simulink model "starshotsim_dev"  (R2023a)
settings: Solver=FixedStepAuto  StartTime=0.0  StopTime=350000  FixedStep=0.01  MaxStep=4.0  MinStep=.001  RelTol=1e-6
values from neighbouring files (symbols this model uses):
  B0 = 3.12e-5    (= 3.12e-05)    [starshot_ACS_setup.m]
  G = 6.67e-11    [starshot_ACS_setup.m]
  M_Earth = 5.972e24    (= 5.972e+24)    [starshot_ACS_setup.m]
  q0 = [qmatlab(2:4),qmatlab(1)]'    [starshot_ACS_setup.m]
  R_Earth = 6.378e6    (= 6378000)    [starshot_ACS_setup.m]
undefined symbols (not defined in the file or in its folder): DiscIntNeverNeededParam, starshot
libraries: simulink x3, dspmathops x3, vrlib x2, sharedtransform x1
(part 1 of 2)
settings Model: SimulationMode=accelerator  Creator=armen  LastModifiedBy=SSDS_1
settings SolverCC: AlgebraicLoopSolver=TrustRegion
settings DataIOCC: ReturnWorkspaceOutputs=off
settings OptimizationCC: DefaultParameterBehavior=Inlined  UseDivisionForNetSlopeComputation=on  UseFloatMulNetSlope=on  InlineInvariantSignals=on  PassReuseOutputArgsAs=Individual arguments  ZeroExternalMemoryAtStartup=off  ZeroInternalMemoryAtStartup=off  NoFixptDivByZeroProtection=on  EfficientFloat2IntCast=on  LifeSpan=1  EfficientTunableParamExpr=on
settings DebuggingCC: ParameterTunabilityLossMsg=error  UnconnectedInputMsg=warning  UnconnectedOutputMsg=warning  UnconnectedLineMsg=warning  ArithmeticOperatorsInVariantConditions=warning
settings HardwareCC: ProdBitPerPointer=32  ProdBitPerSizeT=32  ProdBitPerPtrDiffT=32  ProdLargestAtomicInteger=Long  ProdLargestAtomicFloat=Double  ProdWordSize=32  ProdHWDeviceType=ARM Compatible->ARM Cortex
settings ModelReferenceCC: EnableRefExpFcnMdlSchedulingChecks=on
settings SFSimCC: SimUseLocalCustomCode=off  MATLABDynamicMemAlloc=off  CustomCodeUndefinedFunction=UseInterfaceOnly  SimTargetLang=C++
settings RTWCC: Description=Embedded Coder  SystemTargetFile=ert.tlc  GenCodeOnly=on  TemplateMakefile=ert_default_tmf  GenerateReport=on  RTWUseLocalCustomCode=off  IncludeHyperlinkInReport=on  LaunchReport=on  TargetLang=C++  GenerateTraceInfo=on  GenerateTraceReport=on  GenerateTraceReportSl=on  GenerateTraceReportSf=on  GenerateTraceReportEml=on
settings CodeAppCC: ForceParamTrailComments=on  IgnoreCustomStorageClasses=off  OperatorAnnotations=on  SimulinkDataObjDesc=on  SFDataObjDesc=on  MATLABFcnDesc=on  CustomSymbolStrGlobalVar=rt$N$M  CustomSymbolStrType=$N$M  CustomSymbolStrFcn=$N$M$F  CustomSymbolStrMacro=$N$M  InsertBlockDesc=on  StateflowObjectComments=on  MATLABSourceComments=on
settings ERTTargetCC: TargetLangStandard=C++03 (ISO)  GenerateSampleERTMain=on  IncludeMdlTerminateFcn=off  CombineSignalStateStructs=on  SupportAbsoluteTime=off  CodeInterfacePackaging=C++ class  SupportComplex=off  SupportNonInlinedSFcns=on  InlinedParameterPlacement=NonHierarchical  RootIOFormat=Structure reference  ERTCustomFileTemplate=example_file_process.tlc  ERTFilePackagingFormat=CompactWithDataFile

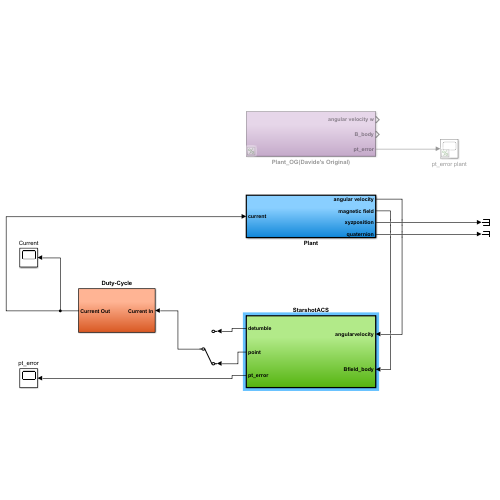
[thumbnail: Simulink's stored preview of the top-level diagram]
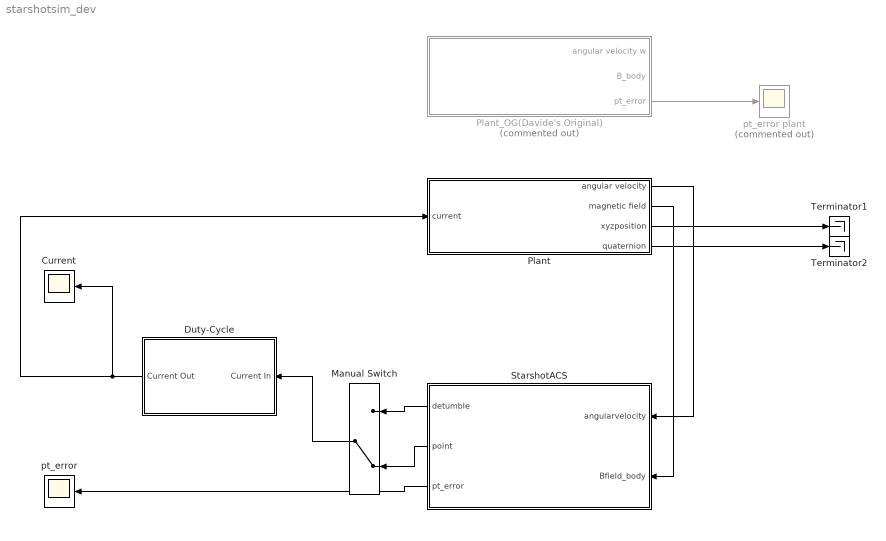
== system starshotsim_dev ==
  Current : Scope
  Duty-Cycle : Subsystem
  Manual Switch : ManualSwitch  CurrentSetting=0
  Plant : Subsystem  TreatAsAtomicUnit=on
  Plant_OG(Davide's Original) : Subsystem  Commented=on
  StarshotACS : Subsystem  TreatAsAtomicUnit=on  SystemSampleTime=0.2
  Terminator1 : Terminator
  Terminator2 : Terminator
  pt_error : Scope
  pt_error plant : Scope  Commented=on
  wires:
  StarshotACS/1(detumble) -> Manual Switch/1
  Plant/4(quaternion) -> Terminator2/1
  Plant/3(xyzposition) -> Terminator1/1
  Plant_OG(Davide's Original)/3(pt_error) -> pt_error plant/1
  StarshotACS/2(point) -> Manual Switch/2
  Plant/1(angular velocity) -> StarshotACS/1(angularvelocity)
  Plant/2(magnetic field) -> StarshotACS/2(Bfield_body)
  Manual Switch/1 -> Duty-Cycle/1(Current In)
  StarshotACS/3(pt_error) -> pt_error/1
  Duty-Cycle/1(Current Out) -> Current/1, Plant/1(current)

== system starshotsim_dev/Duty-Cycle ==
  Current In : Inport
  Demux1 : Demux  Outputs=3
  Duty-cycle input : Constant  Value=starshot.controller.dutyclc
  Mux3 : Mux  Inputs=3
  PWM1 : simulink/Discontinuities/PWM  DisableCoverage=on  Period=starshot.controller.dutyT  InitialDelay=0  DisallowZeroDutyCycle=off  RunAtFixedTimeIntervals=on  SampleTime=0.2
  Product : Product
  Current Out : Outport
  wires:
  Demux1/2 -> Mux3/2
  Demux1/1 -> Mux3/1
  PWM1/1 -> Product/2
  Demux1/3 -> Product/1
  Product/1 -> Mux3/3
  Mux3/1 -> Current Out/1
  Current In/1 -> Demux1/1
  Duty-cycle input/1 -> PWM1/1

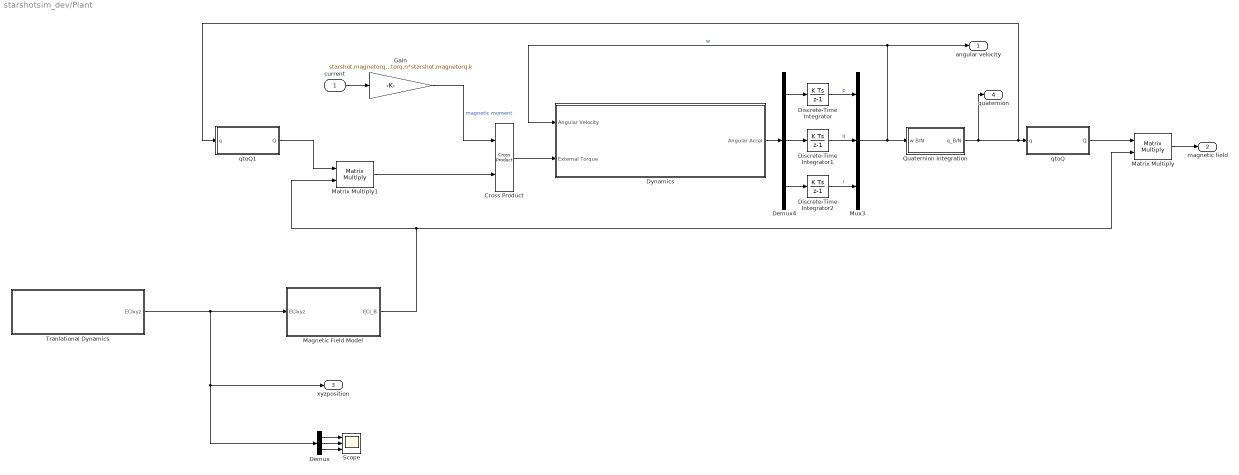
== system starshotsim_dev/Plant ==
  current : Inport
  Cross Product : vrlib/Utilities/Cross Product
  Demux : Demux  Outputs=3
  Demux4 : Demux  Outputs=3
  Discrete-Time Integrator : DiscreteIntegrator  InitialCondition=starshot.IC.w(1)  SampleTime=-1  ICPrevOutput=DiscIntNeverNeededParam  ICPrevScaledInput=DiscIntNeverNeededParam
  Discrete-Time Integrator1 : DiscreteIntegrator  InitialCondition=starshot.IC.w(2)  SampleTime=-1  ICPrevOutput=DiscIntNeverNeededParam  ICPrevScaledInput=DiscIntNeverNeededParam
  Discrete-Time Integrator2 : DiscreteIntegrator  InitialCondition=starshot.IC.w(3)  SampleTime=-1  ICPrevOutput=DiscIntNeverNeededParam  ICPrevScaledInput=DiscIntNeverNeededParam
  Dynamics : Subsystem  TreatAsAtomicUnit=on
  Gain : Gain  Gain=starshot.magnetorq.A*starshot.magnetorq.n*starshot.magnetorq.k
  Magnetic Field Model : Subsystem  TreatAsAtomicUnit=on
  Matrix Multiply : Product  Multiplication=Matrix(*)
  Matrix Multiply1 : Product  Multiplication=Matrix(*)
  Mux3 : Mux  Inputs=3
  Quaternion Integration : Subsystem
  Scope : Scope  NumInputPorts=3
  Tranlational Dynamics : Subsystem  TreatAsAtomicUnit=on
  qtoQ : Subsystem  TreatAsAtomicUnit=on
  qtoQ1 : Subsystem  TreatAsAtomicUnit=on
  angular velocity : Outport
  magnetic field : Outport  Port=2
  xyzposition : Outport  Port=3
  quaternion : Outport  Port=4
  wires:
  Matrix Multiply/1 -> magnetic field/1
  Magnetic Field Model/1(ECI_B) -> Matrix Multiply/2, Matrix Multiply1/2
  Discrete-Time Integrator1/1 -> Mux3/2  "q"
  Discrete-Time Integrator2/1 -> Mux3/3  "r"
  Demux4/3 -> Discrete-Time Integrator2/1
  Demux4/1 -> Discrete-Time Integrator/1
  Tranlational Dynamics/1(ECIxyz) -> Demux/1, xyzposition/1, Magnetic Field Model/1(ECIxyz)
  Quaternion Integration/1(q_B/N) -> qtoQ1/1(q), qtoQ/1(q), quaternion/1
  Dynamics/1(Angular Accel) -> Demux4/1
  Mux3/1 -> Quaternion Integration/1(w B/N), Dynamics/1(Angular Velocity), angular velocity/1  "w"
  current/1 -> Gain/1
  Gain/1 -> Cross Product/1  "magnetic moment"
  Cross Product/1 -> Dynamics/2(External Torque)
  Discrete-Time Integrator/1 -> Mux3/1  "p"
  Demux4/2 -> Discrete-Time Integrator1/1
  Demux/2 -> Scope/2
  Demux/1 -> Scope/1
  Demux/3 -> Scope/3
  qtoQ/1(Q) -> Matrix Multiply/1
  Matrix Multiply1/1 -> Cross Product/2
  qtoQ1/1(Q) -> Matrix Multiply1/1

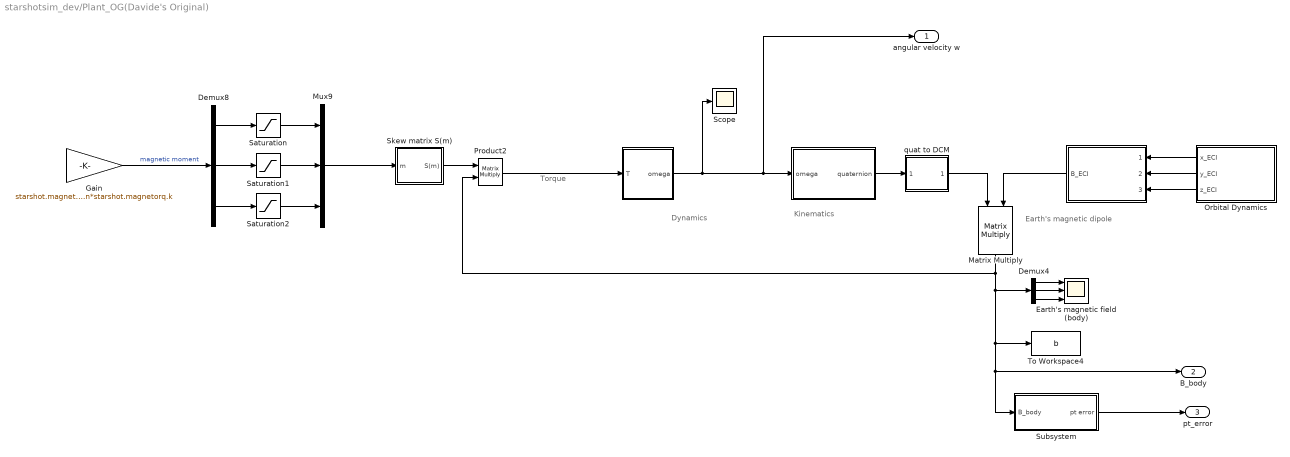
== system starshotsim_dev/Plant_OG(Davide's Original) ==
  note: Torque
  note: Dynamics
  note: Kinematics
  note: Earth's magnetic dipole
  " " : Subsystem
  "   " : Subsystem
  "     " : Subsystem
  Demux4 : Demux  Outputs=3
  Demux8 : Demux  Outputs=3
  Earth's magnetic field (body) : Scope  NumInputPorts=3
  Gain : Gain  Gain=starshot.magnetorq.A*starshot.magnetorq.n*starshot.magnetorq.k
  Matrix Multiply : Product  Multiplication=Matrix(*)
  Mux9 : Mux  Inputs=3
  Orbital Dynamics : Subsystem
  Product2 : Product  Multiplication=Matrix(*)
  Saturation : Saturate  UpperLimit=starshot.magnetorq.m_max_x  LowerLimit=-starshot.magnetorq.m_max_x
  Saturation1 : Saturate  UpperLimit=starshot.magnetorq.m_max_y  LowerLimit=-starshot.magnetorq.m_max_y
  Saturation2 : Saturate  UpperLimit=starshot.magnetorq.m_max_z  LowerLimit=-starshot.magnetorq.m_max_z
  Scope : Scope
  Skew matrix S(m) : Subsystem
  Subsystem : Subsystem
  To Workspace4 : ToWorkspace  VariableName=b  SaveFormat=Timeseries  SampleTime=-1
  quat to DCM : Subsystem  mask(Direction Cosine Matrix){}
      mask help: Determines the 3x3 Direction Cosine Matrix (DCM) from a 4x1 quaternion orientation vector. The outputted DCM transforms vectors from inertial axes to body axes. This version corrects the fucked-up MATLAB one.
      mask Help:
      | <p>This block determines the 3x3 Direction Cosine Matrix (DCM) from a 4x1 quaternion orientation vector. The outputted DCM transforms vectors from inertial axes to body axes.  This version corrects the fucked-up MATLAB one</p>
      | 
      | <p>The block input and output contain more than one signal as described below.</p>
      | 
      | <p><H4>Block Vector Input - Quaternion</H4>
      | <ul>
      | <li>q0</li>
      | <li>q1</li>
      | <li>q2</li>
      | <li>q3</li>
      | </ul>
      | </p>
      | 
      | <p><H4>Block Matrix Output - Direction Cosine Matrix  </H4>
      |     <ul>
      |    </ul>
      |    </p>
      mask Display: disp('q to Q')
  angular velocity w : Outport
  B_body : Outport  Port=2
  pt_error : Outport  Port=3
  wires:
  ? -> Gain/1
  Demux8/2 -> Saturation1/1
  Demux8/1 -> Saturation/1
  Demux8/3 -> Saturation2/1
  Saturation/1 -> Mux9/1
  Saturation1/1 -> Mux9/2
  Saturation2/1 -> Mux9/3
  Mux9/1 -> Skew matrix S(m)/1(m)
  Skew matrix S(m)/1(S(m)) -> Product2/1
  Product2/1 -> "     "/1(T)
  Orbital Dynamics/3(z_ECI) -> " "/3(" ")
  Demux4/3 -> Earth's magnetic field (body)/3
  "   "/1(quaternion) -> quat to DCM/1(e0 e1 e2 e3)
  quat to DCM/1(DCM) -> Matrix Multiply/1
  " "/1(B_ECI) -> Matrix Multiply/2
  Orbital Dynamics/1(x_ECI) -> " "/1(" ")
  Matrix Multiply/1 -> Product2/2, B_body/1, Subsystem/1(B_body), To Workspace4/1, Demux4/1
  Orbital Dynamics/2(y_ECI) -> " "/2(" ")
  Demux4/2 -> Earth's magnetic field (body)/2
  Demux4/1 -> Earth's magnetic field (body)/1
  "     "/1(omega) -> Scope/1, angular velocity w/1, "   "/1(omega)
  Subsystem/1(pt error) -> pt_error/1
  Gain/1 -> Demux8/1  "magnetic moment"

== system starshotsim_dev/StarshotACS ==
  angularvelocity : Inport
  Bfield_body : Inport  Port=2
  KD_controller : Subsystem
  Orientation controller : Subsystem
  Point Error : Subsystem
  detumble : Outport
  point : Outport  Port=2
  pt_error : Outport  Port=3
  wires:
  Bfield_body/1 -> KD_controller/2(B(body)), Point Error/1(B_body), Orientation controller/2(B(body))  "Bfield_body"
  angularvelocity/1 -> Orientation controller/1(Omega), KD_controller/1(Omega)  "angularvelocity"
  Point Error/1(pt error) -> pt_error/1
  KD_controller/1(Current) -> detumble/1
  Orientation controller/1(Current) -> point/1

== system starshotsim_dev/Plant/Dynamics ==
  Angular Velocity : Inport
  External Torque : Inport  Port=2
  Constant : Constant  Value=starshot.IC.massproperties.I
  Constant1 : Constant  Value=starshot.IC.massproperties.Iinv
  Cross Product : vrlib/Utilities/Cross Product
  Product : Product  Multiplication=Matrix(*)
  Product1 : Product  Multiplication=Matrix(*)
  Sum : Sum  Inputs=+-
  Angular Accel : Outport
  wires:
  Angular Velocity/1 -> Cross Product/1, Product/2
  Constant/1 -> Product/1
  Cross Product/1 -> Sum/2
  Product/1 -> Cross Product/2
  External Torque/1 -> Sum/1
  Constant1/1 -> Product1/1
  Product1/1 -> Angular Accel/1
  Sum/1 -> Product1/2

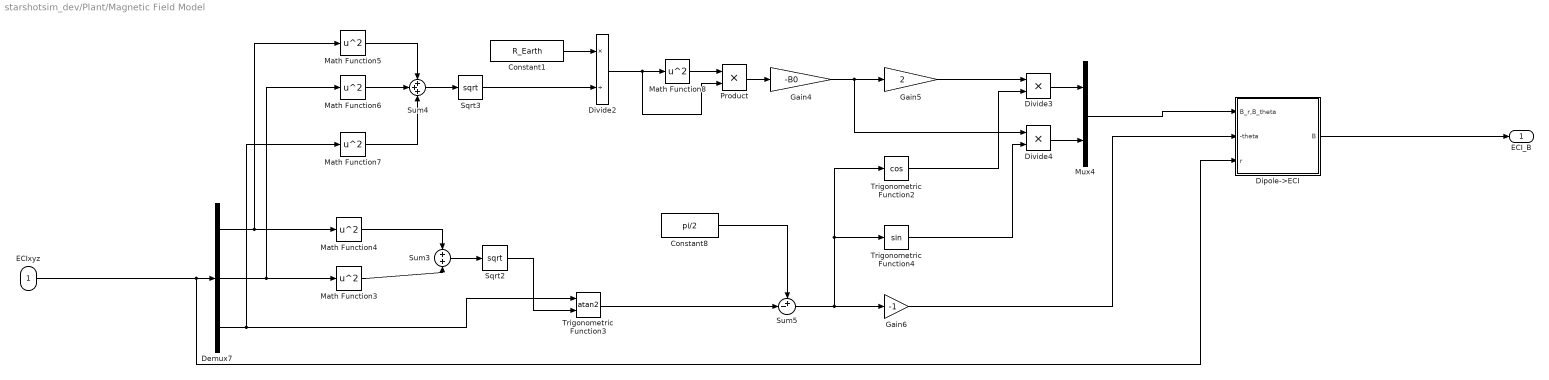
== system starshotsim_dev/Plant/Magnetic Field Model ==
  ECIxyz : Inport
  Constant1 : Constant  Value=R_Earth
  Constant8 : Constant  Value=pi/2
  Demux7 : Demux  Outputs=3
  Dipole->ECI : Subsystem  TreatAsAtomicUnit=on
  Divide2 : Product  Inputs=*/
  Divide3 : Product  Inputs=**
  Divide4 : Product  Inputs=**
  Gain4 : Gain  Gain=-B0
  Gain5 : Gain  Gain=2
  Gain6 : Gain  Gain=-1
  Math Function{3..8} (6 alike) : Math  Operator=square  SignedPower=on
  Mux4 : Mux  Inputs=2
  Product : Product
  Sqrt2 : Sqrt
  Sqrt3 : Sqrt
  Sum3 : Sum
  Sum4 : Sum  Inputs=+++
  Sum5 : Sum  Inputs=+-|
  Trigonometric Function2 : Trigonometry  Operator=cos
  Trigonometric Function3 : Trigonometry  Operator=atan2
  Trigonometric Function4 : Trigonometry
  ECI_B : Outport
  wires:
  Math Function7/1 -> Sum4/3
  Constant1/1 -> Divide2/1
  Math Function5/1 -> Sum4/1
  Math Function4/1 -> Sum3/1
  Demux7/3 -> Math Function7/1, Trigonometric Function3/1
  Sqrt2/1 -> Trigonometric Function3/2
  Product/1 -> Gain4/1
  Math Function8/1 -> Product/1
  Gain5/1 -> Divide3/1
  Sqrt3/1 -> Divide2/2
  Sum4/1 -> Sqrt3/1
  Divide2/1 -> Product/2, Math Function8/1
  Sum3/1 -> Sqrt2/1
  Math Function3/1 -> Sum3/2
  Demux7/1 -> Math Function5/1, Math Function4/1
  Gain4/1 -> Gain5/1, Divide4/1
  Trigonometric Function2/1 -> Divide3/2
  Math Function6/1 -> Sum4/2
  Demux7/2 -> Math Function6/1, Math Function3/1
  Sum5/1 -> Trigonometric Function2/1, Trigonometric Function4/1, Gain6/1
  Trigonometric Function4/1 -> Divide4/2
  Gain6/1 -> Dipole->ECI/2(-theta)
  Divide4/1 -> Mux4/2
  Trigonometric Function3/1 -> Sum5/2
  Constant8/1 -> Sum5/1
  Mux4/1 -> Dipole->ECI/1(B_r,B_theta)
  Dipole->ECI/1(B) -> ECI_B/1
  Divide3/1 -> Mux4/1
  ECIxyz/1 -> Dipole->ECI/3(r), Demux7/1

== system starshotsim_dev/Plant/Quaternion Integration ==
  w B/N : Inport
  Discrete-Time Integrator1 : DiscreteIntegrator  InitialCondition=q0  SampleTime=-1  ICPrevOutput=DiscIntNeverNeededParam  ICPrevScaledInput=DiscIntNeverNeededParam
  q_normalize : Subsystem
  qderiv : Subsystem
  q_B/N : Outport
  wires:
  w B/N/1 -> qderiv/1(w)
  q_normalize/1(q_out) -> qderiv/2(q), q_B/N/1
  Discrete-Time Integrator1/1 -> q_normalize/1(q_in)
  qderiv/1(qd) -> Discrete-Time Integrator1/1

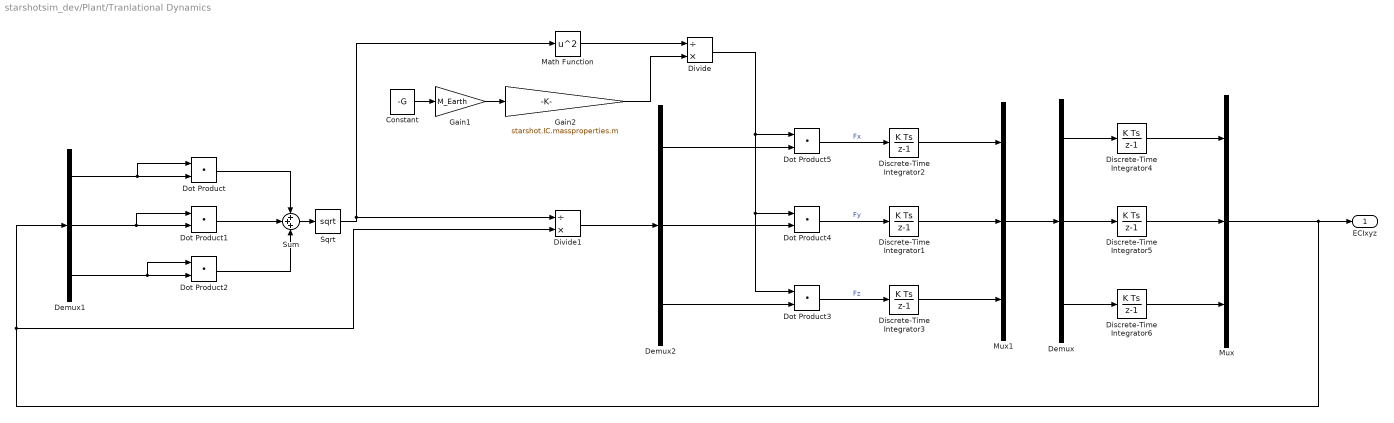
== system starshotsim_dev/Plant/Tranlational Dynamics ==
  Constant : Constant  Value=-G
  Demux : Demux  Outputs=3
  Demux1 : Demux  Outputs=3
  Demux2 : Demux  Outputs=3
  Discrete-Time Integrator1 : DiscreteIntegrator  InitialCondition=starshot.IC.ydot  SampleTime=-1  ICPrevOutput=DiscIntNeverNeededParam  ICPrevScaledInput=DiscIntNeverNeededParam
  Discrete-Time Integrator2 : DiscreteIntegrator  InitialCondition=starshot.IC.xdot  SampleTime=-1  ICPrevOutput=DiscIntNeverNeededParam  ICPrevScaledInput=DiscIntNeverNeededParam
  Discrete-Time Integrator3 : DiscreteIntegrator  InitialCondition=starshot.IC.zdot  SampleTime=-1  ICPrevOutput=DiscIntNeverNeededParam  ICPrevScaledInput=DiscIntNeverNeededParam
  Discrete-Time Integrator4 : DiscreteIntegrator  InitialCondition=starshot.IC.x  SampleTime=-1  ICPrevOutput=DiscIntNeverNeededParam  ICPrevScaledInput=DiscIntNeverNeededParam
  Discrete-Time Integrator5 : DiscreteIntegrator  InitialCondition=starshot.IC.y  SampleTime=-1  ICPrevOutput=DiscIntNeverNeededParam  ICPrevScaledInput=DiscIntNeverNeededParam
  Discrete-Time Integrator6 : DiscreteIntegrator  InitialCondition=starshot.IC.z  SampleTime=-1  ICPrevOutput=DiscIntNeverNeededParam  ICPrevScaledInput=DiscIntNeverNeededParam
  Divide : Product  Inputs=/*
  Divide1 : Product  Inputs=/*
  Dot Product{,1..5} (6 alike) : DotProduct  OutDataTypeStr=Inherit: Inherit via internal rule
  Gain1 : Gain  Gain=M_Earth
  Gain2 : Gain  Gain=starshot.IC.massproperties.m
  Math Function : Math  Operator=square  SignedPower=on
  Mux : Mux  Inputs=3
  Mux1 : Mux  Inputs=3
  Sqrt : Sqrt
  Sum : Sum  Inputs=+++
  ECIxyz : Outport
  wires:
  Discrete-Time Integrator6/1 -> Mux/3
  Discrete-Time Integrator5/1 -> Mux/2
  Discrete-Time Integrator4/1 -> Mux/1
  Demux/3 -> Discrete-Time Integrator6/1
  Demux/1 -> Discrete-Time Integrator4/1
  Mux1/1 -> Demux/1
  Discrete-Time Integrator3/1 -> Mux1/3
  Demux/2 -> Discrete-Time Integrator5/1
  Demux1/2 -> Dot Product1/1, Dot Product1/2
  Sum/1 -> Sqrt/1
  Dot Product4/1 -> Discrete-Time Integrator1/1  "Fy"
  Demux1/1 -> Dot Product/1, Dot Product/2
  Dot Product3/1 -> Discrete-Time Integrator3/1  "Fz"
  Divide/1 -> Dot Product3/1, Dot Product4/1, Dot Product5/1
  Dot Product1/1 -> Sum/2
  Demux1/3 -> Dot Product2/1, Dot Product2/2
  Dot Product2/1 -> Sum/3
  Demux2/2 -> Dot Product4/2
  Demux2/3 -> Dot Product3/2
  Math Function/1 -> Divide/1
  Discrete-Time Integrator1/1 -> Mux1/2
  Gain1/1 -> Gain2/1
  Demux2/1 -> Dot Product5/2
  Dot Product5/1 -> Discrete-Time Integrator2/1  "Fx"
  Dot Product/1 -> Sum/1
  Constant/1 -> Gain1/1
  Divide1/1 -> Demux2/1
  Gain2/1 -> Divide/2
  Sqrt/1 -> Math Function/1, Divide1/1
  Discrete-Time Integrator2/1 -> Mux1/1
  Mux/1 -> ECIxyz/1, Divide1/2, Demux1/1

== system starshotsim_dev/Plant/qtoQ ==
  q : Inport
  Demux : Demux
      settings: DisplayOption=none
  Gain1 : Gain  Gain=2  SaturateOnIntegerOverflow=on  OutDataTypeStr=Inherit: Same as input  ParamDataTypeStr=Inherit: Same as input
  Gain2 : Gain  Gain=2  SaturateOnIntegerOverflow=on  OutDataTypeStr=Inherit: Same as input  ParamDataTypeStr=Inherit: Same as input
  Matrix Gain : Gain  Gain=eye(3,3)  SaturateOnIntegerOverflow=on  OutDataTypeStr=Inherit: Same as input  ParamDataTypeStr=Inherit: Same as input
  Mux : Mux  Inputs=3
  Product : Product  InputSameDT=on  SaturateOnIntegerOverflow=on  OutDataTypeStr=Inherit: Same as first input
  Product1 : Product  InputSameDT=on  SaturateOnIntegerOverflow=on  OutDataTypeStr=Inherit: Same as first input
  Subsystem : Subsystem
      mask Display: disp('3x3 cross matrix')
  Sum1 : Sum  Inputs=|+-  InputSameDT=on  SaturateOnIntegerOverflow=on  OutDataTypeStr=Inherit: Same as first input
  Sum8 : Sum  Inputs=|+-+  InputSameDT=on  SaturateOnIntegerOverflow=on  OutDataTypeStr=Inherit: Same as first input
  T1 : Math  Operator=transpose  SignedPower=on
  T2 : Math  Operator=transpose  SignedPower=on
  qTq : Product  Multiplication=Matrix(*)  InputSameDT=on  SaturateOnIntegerOverflow=on  OutDataTypeStr=Inherit: Same as first input
  qqT : Product  Multiplication=Matrix(*)  InputSameDT=on  SaturateOnIntegerOverflow=on  OutDataTypeStr=Inherit: Same as first input
  Q : Outport
  wires:
  q/1 -> Demux/1
  Demux/1 -> Mux/1
  Matrix Gain/1 -> Sum8/3
  Demux/2 -> Mux/2
  Demux/3 -> Mux/3
  T2/1 -> qTq/1
  Demux/4 -> Product1/2, Product1/1, Product/2
  Product/1 -> Gain1/1
  qqT/1 -> Gain2/1
  Mux/1 -> qTq/2, T2/1, qqT/1, T1/1, Subsystem/1(In1)
  Sum8/1 -> Q/1
  Subsystem/1(Out1) -> Product/1
  Product1/1 -> Sum1/1
  Gain2/1 -> Sum8/1
  T1/1 -> qqT/2
  Gain1/1 -> Sum8/2
  qTq/1 -> Sum1/2
  Sum1/1 -> Matrix Gain/1

== system starshotsim_dev/Plant/qtoQ1 ==
  q : Inport
  Demux : Demux
      settings: DisplayOption=none
  Gain1 : Gain  Gain=2  SaturateOnIntegerOverflow=on  OutDataTypeStr=Inherit: Same as input  ParamDataTypeStr=Inherit: Same as input
  Gain2 : Gain  Gain=2  SaturateOnIntegerOverflow=on  OutDataTypeStr=Inherit: Same as input  ParamDataTypeStr=Inherit: Same as input
  Matrix Gain : Gain  Gain=eye(3,3)  SaturateOnIntegerOverflow=on  OutDataTypeStr=Inherit: Same as input  ParamDataTypeStr=Inherit: Same as input
  Mux : Mux  Inputs=3
  Product : Product  InputSameDT=on  SaturateOnIntegerOverflow=on  OutDataTypeStr=Inherit: Same as first input
  Product1 : Product  InputSameDT=on  SaturateOnIntegerOverflow=on  OutDataTypeStr=Inherit: Same as first input
  Subsystem : Subsystem
      mask Display: disp('3x3 cross matrix')
  Sum1 : Sum  Inputs=|+-  InputSameDT=on  SaturateOnIntegerOverflow=on  OutDataTypeStr=Inherit: Same as first input
  Sum8 : Sum  Inputs=|+-+  InputSameDT=on  SaturateOnIntegerOverflow=on  OutDataTypeStr=Inherit: Same as first input
  T1 : Math  Operator=transpose  SignedPower=on
  T2 : Math  Operator=transpose  SignedPower=on
  qTq : Product  Multiplication=Matrix(*)  InputSameDT=on  SaturateOnIntegerOverflow=on  OutDataTypeStr=Inherit: Same as first input
  qqT : Product  Multiplication=Matrix(*)  InputSameDT=on  SaturateOnIntegerOverflow=on  OutDataTypeStr=Inherit: Same as first input
  Q : Outport
  wires:
  Sum1/1 -> Matrix Gain/1
  qTq/1 -> Sum1/2
  Gain1/1 -> Sum8/2
  T1/1 -> qqT/2
  Gain2/1 -> Sum8/1
  Product1/1 -> Sum1/1
  Subsystem/1(Out1) -> Product/1
  Sum8/1 -> Q/1
  Mux/1 -> Subsystem/1(In1), T1/1, qqT/1, T2/1, qTq/2
  qqT/1 -> Gain2/1
  Product/1 -> Gain1/1
  Demux/4 -> Product/2, Product1/1, Product1/2
  T2/1 -> qTq/1
  Demux/3 -> Mux/3
  Demux/2 -> Mux/2
  Matrix Gain/1 -> Sum8/3
  Demux/1 -> Mux/1
  q/1 -> Demux/1

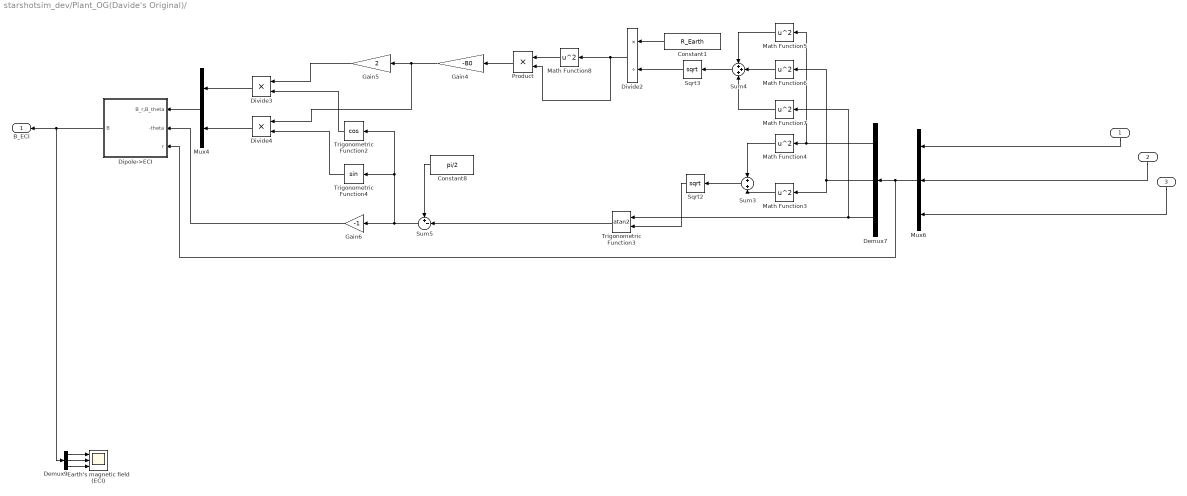
== system starshotsim_dev/Plant_OG(Davide's Original)/  ==
  " " : Inport
  " " : Inport  Port=2
  " " : Inport  Port=3
  Constant1 : Constant  Value=R_Earth
  Constant8 : Constant  Value=pi/2
  Demux7 : Demux  Outputs=3
  Demux9 : Demux  Outputs=3
  Dipole->ECI : Subsystem
  Divide2 : Product  Inputs=*/
  Divide3 : Product  Inputs=**
  Divide4 : Product  Inputs=**
  Earth's magnetic field (ECI) : Scope  NumInputPorts=3
  Gain4 : Gain  Gain=-B0
  Gain5 : Gain  Gain=2
  Gain6 : Gain  Gain=-1
  Math Function{3..8} (6 alike) : Math  Operator=square  SignedPower=on
  Mux4 : Mux  Inputs=2
  Mux6 : Mux  Inputs=3
  Product : Product
  Sqrt2 : Sqrt
  Sqrt3 : Sqrt
  Sum3 : Sum
  Sum4 : Sum  Inputs=+++
  Sum5 : Sum  Inputs=+-|
  Trigonometric Function2 : Trigonometry  Operator=cos
  Trigonometric Function3 : Trigonometry  Operator=atan2
  Trigonometric Function4 : Trigonometry
  B_ECI : Outport
  wires:
  Math Function6/1 -> Sum4/2
  Math Function5/1 -> Sum4/1
  Math Function7/1 -> Sum4/3
  Sum4/1 -> Sqrt3/1
  Sqrt3/1 -> Divide2/2
  Constant1/1 -> Divide2/1
  Trigonometric Function2/1 -> Divide3/2
  Trigonometric Function4/1 -> Divide4/2
  Divide3/1 -> Mux4/1
  Divide4/1 -> Mux4/2
  Mux4/1 -> Dipole->ECI/1(B_r,B_theta)
  Gain6/1 -> Dipole->ECI/2(-theta)
  Sum5/1 -> Trigonometric Function2/1, Trigonometric Function4/1, Gain6/1
  Demux7/1 -> Math Function5/1, Math Function4/1
  Divide2/1 -> Product/2, Math Function8/1
  Math Function8/1 -> Product/1
  Product/1 -> Gain4/1
  Gain4/1 -> Divide4/1, Gain5/1
  Gain5/1 -> Divide3/1
  Mux6/1 -> Dipole->ECI/3(r), Demux7/1
  Trigonometric Function3/1 -> Sum5/2
  Sqrt2/1 -> Trigonometric Function3/2
  " "/1 -> Mux6/1
  Math Function4/1 -> Sum3/1
  Math Function3/1 -> Sum3/2
  Sum3/1 -> Sqrt2/1
  Demux7/3 -> Math Function7/1, Trigonometric Function3/1
  Demux7/2 -> Math Function3/1, Math Function6/1
  Constant8/1 -> Sum5/1
  " "/1 -> Mux6/2
  " "/1 -> Mux6/3
  Demux9/2 -> Earth's magnetic field (ECI)/2
  Demux9/3 -> Earth's magnetic field (ECI)/3
  Demux9/1 -> Earth's magnetic field (ECI)/1
  Dipole->ECI/1(B) -> Demux9/1, B_ECI/1

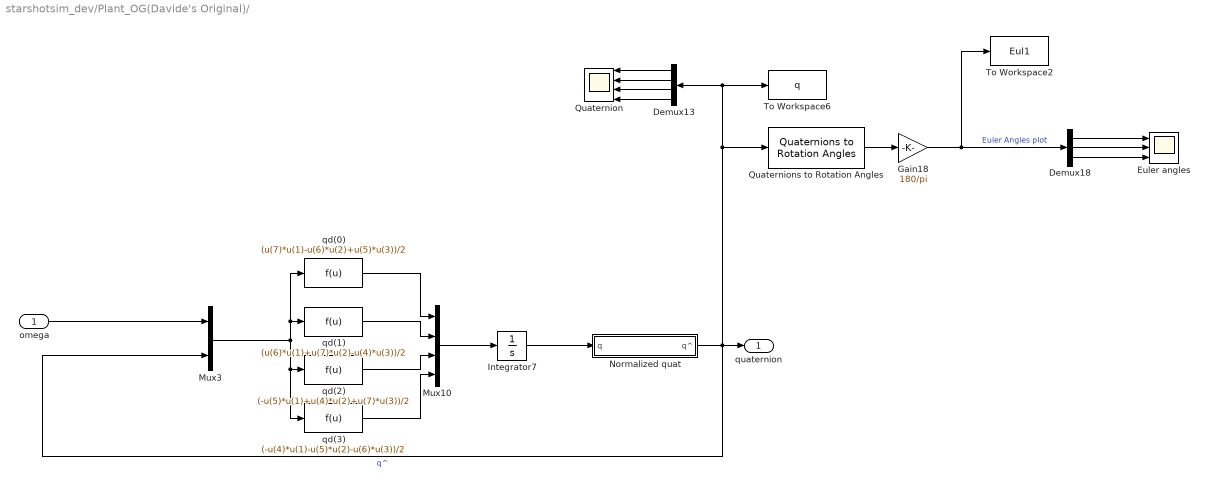
== system starshotsim_dev/Plant_OG(Davide's Original)/    ==
  omega : Inport
  Demux13 : Demux
  Demux18 : Demux  Outputs=3
  Euler angles : Scope  NumInputPorts=3
  Gain18 : Gain  Gain=180/pi
  Integrator7 : Integrator  InitialCondition=q0
  Mux10 : Mux
  Mux3 : Mux  Inputs=2
  Normalized quat : Subsystem
  Quaternion : Scope  NumInputPorts=4
  Quaternions to Rotation Angles : sharedtransform/Quaternions to Rotation Angles  rotationOrder=ZYX  aMode=aMode
  To Workspace2 : ToWorkspace  VariableName=Eul1  SaveFormat=Timeseries  SampleTime=-1
  To Workspace6 : ToWorkspace  VariableName=q  SaveFormat=Timeseries  SampleTime=-1
  qd(0) : Fcn  Expr=(u(7)*u(1)-u(6)*u(2)+u(5)*u(3))/2
  qd(1) : Fcn  Expr=(u(6)*u(1)+u(7)*u(2)-u(4)*u(3))/2
  qd(2) : Fcn  Expr=(-u(5)*u(1)+u(4)*u(2)+u(7)*u(3))/2
  qd(3) : Fcn  Expr=(-u(4)*u(1)-u(5)*u(2)-u(6)*u(3))/2
  quaternion : Outport
  wires:
  qd(2)/1 -> Mux10/3
  Normalized quat/1(q^) -> Mux3/2, Quaternions to Rotation Angles/1, To Workspace6/1, Demux13/1, quaternion/1  "q^"
  omega/1 -> Mux3/1
  qd(1)/1 -> Mux10/2
  qd(3)/1 -> Mux10/4
  Integrator7/1 -> Normalized quat/1(q)
  Mux10/1 -> Integrator7/1
  qd(0)/1 -> Mux10/1
  Mux3/1 -> qd(3)/1, qd(2)/1, qd(1)/1, qd(0)/1
  Demux13/1 -> Quaternion/1
  Demux18/1 -> Euler angles/1
  Demux18/3 -> Euler angles/3
  Gain18/1 -> To Workspace2/1, Demux18/1  "Euler Angles plot"
  Demux13/4 -> Quaternion/4
  Demux18/2 -> Euler angles/2
  Demux13/3 -> Quaternion/3
  Quaternions to Rotation Angles/1 -> Gain18/1
  Demux13/2 -> Quaternion/2

== system starshotsim_dev/Plant_OG(Davide's Original)/      ==
  T : Inport
  (w_b)x(L_b) : Subsystem
  Angular velocity : Scope  NumInputPorts=3
  Demux16 : Demux  Outputs=3
  Integrator6 : Integrator  InitialCondition=starshot.IC.w
  Inv(I) : Gain  Gain=starshot.IC.massproperties.Iinv  Multiplication=Matrix(K*u)
  Sum12 : Sum  Inputs=|+-
  To Workspace1 : ToWorkspace  VariableName=w  SaveFormat=Timeseries  SampleTime=-1
  XY Graph : Record  FileSettingsInternal="{\"entries\":[{\"content\":{\"excelSettings\":{\"content\":{},\"type\":\"Streamout.ExcelSettings\"}},\"type\":\"Streamout.FileSettingStorage\",\"uuid\":\"\"}],\"packageUris\":[\"http:\\/\\/schema.mathworks.com\\/mf0\\/streamout_blocks\\/R2020a\"],\"version\":\"1.0\"}"  Layout=[1 1]  SignalsInternal="{\"entries\":[{\"content\":{\"signals\":[{\"content\":{\"blockPath\":[],\"dimensions\":[1],\"domain\":\"\",\"lineColor\":\"#a2142f\",\"plots\":[1],\"port\":1,\"signalID\":19233,\"signalName\":\"Demux16:1\"},\"type\":\"RecordBlkView.Signal\",\"uuid\":\"\"},{\"content\":{\"blockPath\":[],\"dimensions\":[1],\"domain\":\"\",\"lineColor\":\"#139fff\",\"plots\":[1],\"port\":2,\"signalID\":19236,\"signalName\":\"Demux16:2\"},\"type\":\"RecordBlkView.Signal\",\"uuid\":\"\"}]},\"type\":\"RecordBlkView.InputSignals\",\"uuid\":\"\"}],\"packageUris\":[\"http:\\/\\/schema.mathworks.com\\/mf0\\/streamout_blocks\\/R2020a\"],\"version\":\"1.0\"}"  VisualizationBindings="{\"xyplotplugin\":{\"info\":[{\"series\":[{\"bindingParametersList\":[{\"parameter\":\"X-Axis\",\"signalID\":19233,\"signalName\":\"Demux16:1\"},{\"parameter\":\"Y-Axis\",\"signalID\":19236,\"signalName\":\"Demux16:2\"}],\"seriesID\":49118}],\"subplotID\":1}]}}"  CompatibilityTag=XY  st=-1
  omega : Outport
  wires:
  Inv(I)/1 -> Integrator6/1
  Integrator6/1 -> Demux16/1, To Workspace1/1, omega/1, (w_b)x(L_b)/2(L_b), (w_b)x(L_b)/1(w_b)  "w"
  (w_b)x(L_b)/1((w_b)x(L_b)) -> Sum12/2
  Sum12/1 -> Inv(I)/1  "wdot"
  T/1 -> Sum12/1
  Demux16/1 -> XY Graph/1, Angular velocity/1
  Demux16/2 -> XY Graph/2, Angular velocity/2
  Demux16/3 -> Angular velocity/3

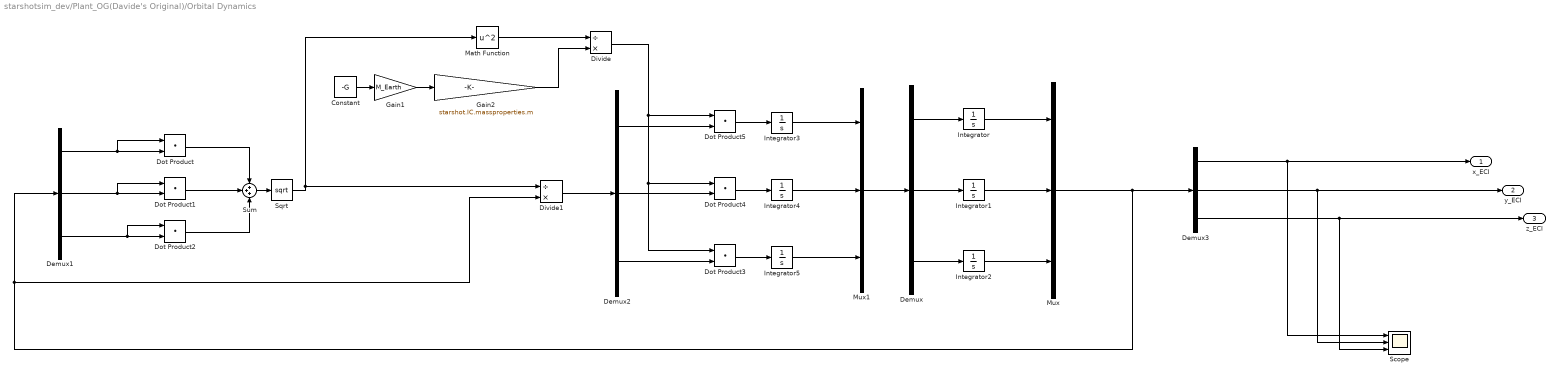
== system starshotsim_dev/Plant_OG(Davide's Original)/Orbital Dynamics ==
  Constant : Constant  Value=-G
  Demux{,1..3} (4 alike) : Demux  Outputs=3
  Divide : Product  Inputs=/*
  Divide1 : Product  Inputs=/*
  Dot Product{,1..5} (6 alike) : DotProduct  OutDataTypeStr=Inherit: Inherit via internal rule
  Gain1 : Gain  Gain=M_Earth
  Gain2 : Gain  Gain=starshot.IC.massproperties.m
  Integrator : Integrator  InitialCondition=starshot.IC.x
  Integrator1 : Integrator  InitialCondition=starshot.IC.y
  Integrator2 : Integrator  InitialCondition=starshot.IC.z
  Integrator3 : Integrator  InitialCondition=starshot.IC.xdot
  Integrator4 : Integrator  InitialCondition=starshot.IC.ydot
  Integrator5 : Integrator  InitialCondition=starshot.IC.zdot
  Math Function : Math  Operator=square  SignedPower=on
  Mux : Mux  Inputs=3
  Mux1 : Mux  Inputs=3
  Scope : Scope  NumInputPorts=3
  Sqrt : Sqrt
  Sum : Sum  Inputs=+++
  x_ECI : Outport
  y_ECI : Outport  Port=2
  z_ECI : Outport  Port=3
  wires:
  Integrator/1 -> Mux/1
  Integrator2/1 -> Mux/3
  Integrator1/1 -> Mux/2
  Demux/3 -> Integrator2/1
  Demux/2 -> Integrator1/1
  Demux/1 -> Integrator/1
  Mux1/1 -> Demux/1
  Integrator5/1 -> Mux1/3
  Integrator4/1 -> Mux1/2
  Constant/1 -> Gain1/1
  Integrator3/1 -> Mux1/1
  Demux1/1 -> Dot Product/1, Dot Product/2
  Demux1/2 -> Dot Product1/1, Dot Product1/2
  Demux1/3 -> Dot Product2/1, Dot Product2/2
  Dot Product1/1 -> Sum/2
  Dot Product2/1 -> Sum/3
  Dot Product/1 -> Sum/1
  Sum/1 -> Sqrt/1
  Sqrt/1 -> Math Function/1, Divide1/1
  Gain1/1 -> Gain2/1
  Divide/1 -> Dot Product3/1, Dot Product4/1, Dot Product5/1
  Dot Product5/1 -> Integrator3/1
  Dot Product4/1 -> Integrator4/1
  Gain2/1 -> Divide/2
  Math Function/1 -> Divide/1
  Demux2/3 -> Dot Product3/2
  Demux2/2 -> Dot Product4/2
  Demux2/1 -> Dot Product5/2
  Dot Product3/1 -> Integrator5/1
  Divide1/1 -> Demux2/1
  Mux/1 -> Divide1/2, Demux1/1, Demux3/1
  Demux3/3 -> Scope/3, z_ECI/1
  Demux3/2 -> Scope/2, y_ECI/1
  Demux3/1 -> Scope/1, x_ECI/1

== system starshotsim_dev/Plant_OG(Davide's Original)/Skew matrix S(m) ==
  m : Inport
  Constant3 : Constant  Value=0
  Demux : Demux  Outputs=3
  Gain : Gain  Gain=-1
  Gain1 : Gain  Gain=-1
  Gain2 : Gain  Gain=-1
  Mux : Mux  Inputs=3
  Mux1 : Mux  Inputs=3
  Mux2 : Mux  Inputs=3
  Vector Concatenate : Concatenate  NumInputs=3  Mode=Multidimensional array  ConcatenateDimension=2
  S(m) : Outport
  wires:
  Gain/1 -> Mux/3
  Demux/2 -> Mux2/1, Gain/1
  Demux/3 -> Gain1/1, Mux/2
  Gain2/1 -> Mux2/2
  Demux/1 -> Mux1/3, Gain2/1
  Mux1/1 -> Vector Concatenate/2
  m/1 -> Demux/1
  Constant3/1 -> Mux2/3, Mux/1, Mux1/2
  Vector Concatenate/1 -> S(m)/1
  Mux/1 -> Vector Concatenate/1
  Mux2/1 -> Vector Concatenate/3
  Gain1/1 -> Mux1/1

== system starshotsim_dev/Plant_OG(Davide's Original)/Subsystem ==
  B_body : Inport
  Acos : Trigonometry  Operator=acos
  Constant : Constant  Value=[0,0,1]
  Dot Product : DotProduct  OutDataTypeStr=Inherit: Inherit via internal rule
  Multiply : Gain  Gain=180/pi
  Normalization : dspmathops/Normalization  NormType=2-norm  Bias=1e-10  NormOver=Each column  Dimension=1  roundingMode=Floor  overflowMode=off  accumDataTypeStr=Inherit: Same as product output  accumLastDataTypeStr=Inherit: Same as product output  outputDataTypeStr=Inherit: Same as product output  outputMin=[]  outputMax=[]  outputLastDataTypeStr=Inherit: Same as product output
  Saturation3 : Saturate  UpperLimit=1  LowerLimit=-1
  pt error : Outport
  wires:
  Saturation3/1 -> Acos/1
  Normalization/1 -> Dot Product/1
  Dot Product/1 -> Saturation3/1
  Constant/1 -> Dot Product/2
  Acos/1 -> Multiply/1
  B_body/1 -> Normalization/1
  Multiply/1 -> pt error/1

== system starshotsim_dev/Plant_OG(Davide's Original)/quat to DCM ==
  e0 e1 e2 e3 : Inport
  Demux : Demux
      settings: DisplayOption=none
  Gain1 : Gain  Gain=2  SaturateOnIntegerOverflow=on  OutDataTypeStr=Inherit: Same as input  ParamDataTypeStr=Inherit: Same as input
  Gain2 : Gain  Gain=2  SaturateOnIntegerOverflow=on  OutDataTypeStr=Inherit: Same as input  ParamDataTypeStr=Inherit: Same as input
  Matrix Gain : Gain  Gain=eye(3,3)  SaturateOnIntegerOverflow=on  OutDataTypeStr=Inherit: Same as input  ParamDataTypeStr=Inherit: Same as input
  Mux : Mux  Inputs=3
  Product : Product  InputSameDT=on  SaturateOnIntegerOverflow=on  OutDataTypeStr=Inherit: Same as first input
  Product1 : Product  InputSameDT=on  SaturateOnIntegerOverflow=on  OutDataTypeStr=Inherit: Same as first input
  Subsystem : Subsystem
      mask Display: disp('3x3 cross matrix')
  Sum1 : Sum  Inputs=|+-  InputSameDT=on  SaturateOnIntegerOverflow=on  OutDataTypeStr=Inherit: Same as first input
  Sum8 : Sum  Inputs=|+-+  InputSameDT=on  SaturateOnIntegerOverflow=on  OutDataTypeStr=Inherit: Same as first input
  T1 : Math  Operator=transpose  SignedPower=on
  T2 : Math  Operator=transpose  SignedPower=on
  qTq : Product  Multiplication=Matrix(*)  InputSameDT=on  SaturateOnIntegerOverflow=on  OutDataTypeStr=Inherit: Same as first input
  qqT : Product  Multiplication=Matrix(*)  InputSameDT=on  SaturateOnIntegerOverflow=on  OutDataTypeStr=Inherit: Same as first input
  DCM : Outport  InitialOutput=0
  wires:
  Subsystem/1(Out1) -> Product/1
  Matrix Gain/1 -> Sum8/3
  Sum1/1 -> Matrix Gain/1
  qTq/1 -> Sum1/2
  T2/1 -> qTq/1
  Product1/1 -> Sum1/1
  Gain1/1 -> Sum8/2
  Gain2/1 -> Sum8/1
  qqT/1 -> Gain2/1
  T1/1 -> qqT/2
  Product/1 -> Gain1/1
  Mux/1 -> qTq/2, T2/1, qqT/1, T1/1, Subsystem/1(In1)
  Demux/4 -> Product1/2, Product1/1, Product/2
  Demux/3 -> Mux/3
  Demux/2 -> Mux/2
  Demux/1 -> Mux/1
  e0 e1 e2 e3/1 -> Demux/1
  Sum8/1 -> DCM/1

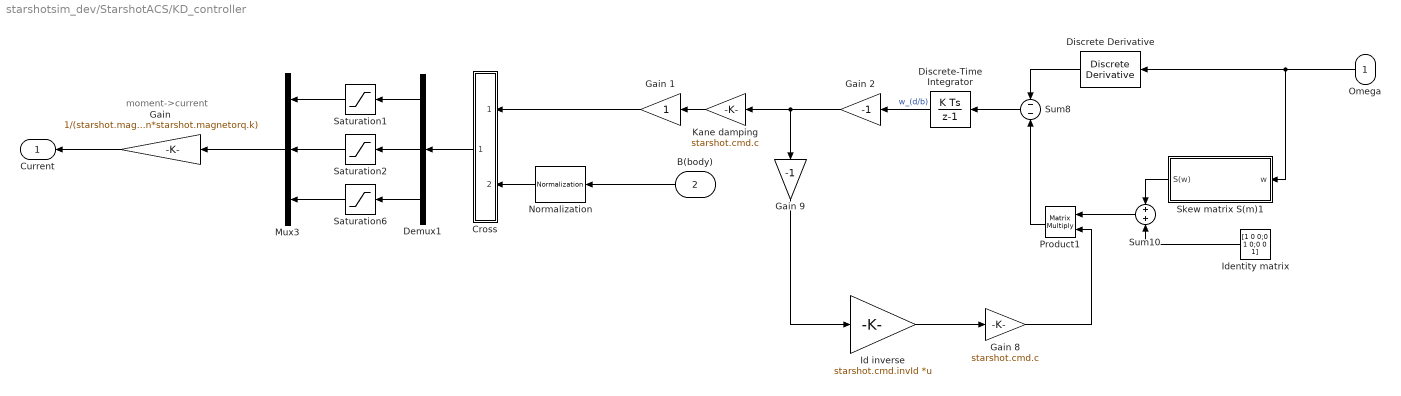
== system starshotsim_dev/StarshotACS/KD_controller ==
  note: moment->current
  Omega : Inport
  B(body) : Inport  Port=2
  Cross : Subsystem
  Demux1 : Demux  Outputs=3
  Discrete Derivative : simulink/Discrete/Discrete Derivative  gainval=1.0  ICPrevScaledInput=0.0  OutMin=[]  OutMax=[]  OutDataType=fixdt(1, 16)  OutScaling=2^-10  DoSatur=off
  Discrete-Time Integrator : DiscreteIntegrator  InitialCondition=starshot.cmd.wdb0  SampleTime=-1  ICPrevOutput=DiscIntNeverNeededParam  ICPrevScaledInput=DiscIntNeverNeededParam
  Gain : Gain  Gain=1/(starshot.magnetorq.A*starshot.magnetorq.n*starshot.magnetorq.k)
  Gain 1 : Gain  SaturateOnIntegerOverflow=on  OutDataTypeStr=Inherit: Same as input  ParamDataTypeStr=Inherit: Same as input
  Gain 2 : Gain  Gain=-1  SaturateOnIntegerOverflow=on  OutDataTypeStr=Inherit: Same as input  ParamDataTypeStr=Inherit: Same as input
  Gain 8 : Gain  Gain=starshot.cmd.c  SaturateOnIntegerOverflow=on  OutDataTypeStr=Inherit: Same as input  ParamDataTypeStr=Inherit: Same as input
  Gain 9 : Gain  Gain=-1  SaturateOnIntegerOverflow=on  OutDataTypeStr=Inherit: Same as input  ParamDataTypeStr=Inherit: Same as input
  Id inverse : Gain  Gain=starshot.cmd.invId  Multiplication=Matrix(K*u)  SaturateOnIntegerOverflow=on  OutDataTypeStr=Inherit: Same as input  ParamDataTypeStr=Inherit: Same as input
  Identity matrix : Constant  Value=[1 0 0;0 1 0;0 0 1]
  Kane damping : Gain  Gain=starshot.cmd.c  SaturateOnIntegerOverflow=on  OutDataTypeStr=Inherit: Same as input  ParamDataTypeStr=Inherit: Same as input
  Mux3 : Mux  Inputs=3
  Normalization : dspmathops/Normalization  NormType=Squared 2-norm  Bias=1e-10  NormOver=Each column  Dimension=1  roundingMode=Floor  overflowMode=off  accumDataTypeStr=Inherit: Same as product output  accumLastDataTypeStr=Inherit: Same as product output  outputDataTypeStr=Inherit: Same as product output  outputMin=[]  outputMax=[]  outputLastDataTypeStr=Inherit: Same as product output
  Product1 : Product  Multiplication=Matrix(*)
  Saturation1 : Saturate  UpperLimit=starshot.magnetorq.m_max_x  LowerLimit=-starshot.magnetorq.m_max_x
  Saturation2 : Saturate  UpperLimit=starshot.magnetorq.m_max_y  LowerLimit=-starshot.magnetorq.m_max_y
  Saturation6 : Saturate  UpperLimit=starshot.magnetorq.m_max_z  LowerLimit=-starshot.magnetorq.m_max_z
  Skew matrix S(m)1 : Subsystem
  Sum10 : Sum  Inputs=+|+  InputSameDT=on  SaturateOnIntegerOverflow=on  OutDataTypeStr=Inherit: Same as first input
  Sum8 : Sum  Inputs=--
  Current : Outport
  wires:
  Discrete-Time Integrator/1 -> Gain 2/1  "w_(d/b)"
  Omega/1 -> Discrete Derivative/1, Skew matrix S(m)1/1(w)
  B(body)/1 -> Normalization/1
  Gain 2/1 -> Kane damping/1, Gain 9/1
  Normalization/1 -> Cross/2(B)
  Kane damping/1 -> Gain 1/1
  Discrete Derivative/1 -> Sum8/1
  Sum8/1 -> Discrete-Time Integrator/1
  Gain 8/1 -> Product1/2
  Id inverse/1 -> Gain 8/1
  Skew matrix S(m)1/1(S(w)) -> Sum10/1
  Identity matrix/1 -> Sum10/2
  Gain 9/1 -> Id inverse/1
  Sum10/1 -> Product1/1
  Product1/1 -> Sum8/2
  Gain 1/1 -> Cross/1(A)
  Gain/1 -> Current/1
  Cross/1(AxB) -> Demux1/1
  Saturation1/1 -> Mux3/1
  Mux3/1 -> Gain/1
  Demux1/1 -> Saturation1/1
  Demux1/2 -> Saturation2/1
  Saturation6/1 -> Mux3/3
  Demux1/3 -> Saturation6/1
  Saturation2/1 -> Mux3/2

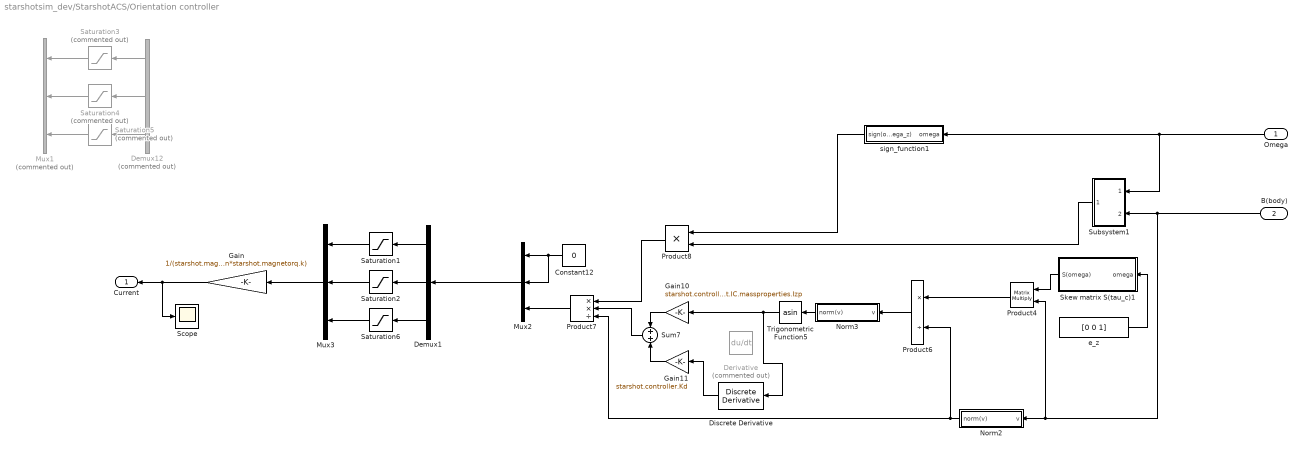
== system starshotsim_dev/StarshotACS/Orientation controller ==
  Omega : Inport
  B(body) : Inport  Port=2
  Constant12 : Constant  Value=0
  Demux1 : Demux  Outputs=3
  Demux12 : Demux  Commented=on  Outputs=3
  Derivative : Derivative  Commented=on
  Discrete Derivative : simulink/Discrete/Discrete Derivative  gainval=1.0  ICPrevScaledInput=0.0  OutMin=[]  OutMax=[]  OutDataType=fixdt(1, 16)  OutScaling=2^-10  DoSatur=off
  Gain : Gain  Gain=1/(starshot.magnetorq.A*starshot.magnetorq.n*starshot.magnetorq.k)
  Gain10 : Gain  Gain=starshot.controller.Kp*starshot.IC.massproperties.Izp
  Gain11 : Gain  Gain=starshot.controller.Kd
  Mux1 : Mux  Commented=on  Inputs=3
  Mux2 : Mux  Inputs=3
  Mux3 : Mux  Inputs=3
  Norm2 : Subsystem
  Norm3 : Subsystem
  Product4 : Product  Multiplication=Matrix(*)
  Product6 : Product  Inputs=*/
  Product7 : Product  Inputs=**/
  Product8 : Product  Inputs=**
  Saturation1 : Saturate  UpperLimit=starshot.magnetorq.m_max_x  LowerLimit=-starshot.magnetorq.m_max_x
  Saturation2 : Saturate  UpperLimit=starshot.magnetorq.m_max_y  LowerLimit=-starshot.magnetorq.m_max_y
  Saturation3 : Saturate  Commented=on  UpperLimit=0.250  LowerLimit=-0.250
  Saturation4 : Saturate  Commented=on  UpperLimit=0.250  LowerLimit=-0.250
  Saturation5 : Saturate  Commented=on  UpperLimit=0.250  LowerLimit=-0.250
  Saturation6 : Saturate  UpperLimit=starshot.magnetorq.m_max_z  LowerLimit=-starshot.magnetorq.m_max_z
  Scope : Scope
  Skew matrix S(tau_c)1 : Subsystem
  Subsystem1 : Subsystem
  Sum7 : Sum  Inputs=+|+
  Trigonometric Function5 : Trigonometry  Operator=asin
  e_z : Constant  Value=[0 0 1]
  sign_function1 : Subsystem
  Current : Outport
  wires:
  Product4/1 -> Product6/1
  Sum7/1 -> Product7/2
  Trigonometric Function5/1 -> Discrete Derivative/1, Gain10/1
  Norm3/1(norm(v)) -> Trigonometric Function5/1
  e_z/1 -> Skew matrix S(tau_c)1/1(omega)
  Product7/1 -> Mux2/3
  Constant12/1 -> Mux2/2, Mux2/1
  Skew matrix S(tau_c)1/1(S(omega)) -> Product4/1
  Norm2/1(norm(v)) -> Product7/3, Product6/2
  Gain10/1 -> Sum7/1
  Product6/1 -> Norm3/1(v)
  Product8/1 -> Product7/1
  Gain11/1 -> Sum7/2
  B(body)/1 -> Product4/2, Norm2/1(v), Subsystem1/2(B(body))
  sign_function1/1(sign(omega_z)) -> Product8/1
  Subsystem1/1(sign(cos)) -> Product8/2
  Omega/1 -> Subsystem1/1(omega), sign_function1/1(omega)
  Demux12/1 -> Saturation3/1
  Saturation3/1 -> Mux1/1
  Saturation5/1 -> Mux1/3
  Demux12/2 -> Saturation4/1
  Saturation4/1 -> Mux1/2
  Demux12/3 -> Saturation5/1
  Demux1/3 -> Saturation6/1
  Saturation6/1 -> Mux3/3
  Demux1/2 -> Saturation2/1
  Saturation2/1 -> Mux3/2
  Demux1/1 -> Saturation1/1
  Saturation1/1 -> Mux3/1
  Gain/1 -> Scope/1, Current/1
  Mux3/1 -> Gain/1
  Mux2/1 -> Demux1/1
  Discrete Derivative/1 -> Gain11/1

== system starshotsim_dev/StarshotACS/Point Error ==
  B_body : Inport
  Acos : Trigonometry  Operator=acos
  Constant : Constant  Value=[0,0,1]
  Dot Product : DotProduct  OutDataTypeStr=Inherit: Inherit via internal rule
  Multiply : Gain  Gain=180/pi
  Normalization : dspmathops/Normalization  NormType=2-norm  Bias=1e-10  NormOver=Each column  Dimension=1  roundingMode=Floor  overflowMode=off  accumDataTypeStr=Inherit: Same as product output  accumLastDataTypeStr=Inherit: Same as product output  outputDataTypeStr=Inherit: Same as product output  outputMin=[]  outputMax=[]  outputLastDataTypeStr=Inherit: Same as product output
  Saturation3 : Saturate  UpperLimit=1  LowerLimit=-1
  pt error : Outport
  wires:
  Saturation3/1 -> Acos/1
  Normalization/1 -> Dot Product/1
  Dot Product/1 -> Saturation3/1
  Constant/1 -> Dot Product/2
  Acos/1 -> Multiply/1
  B_body/1 -> Normalization/1
  Multiply/1 -> pt error/1

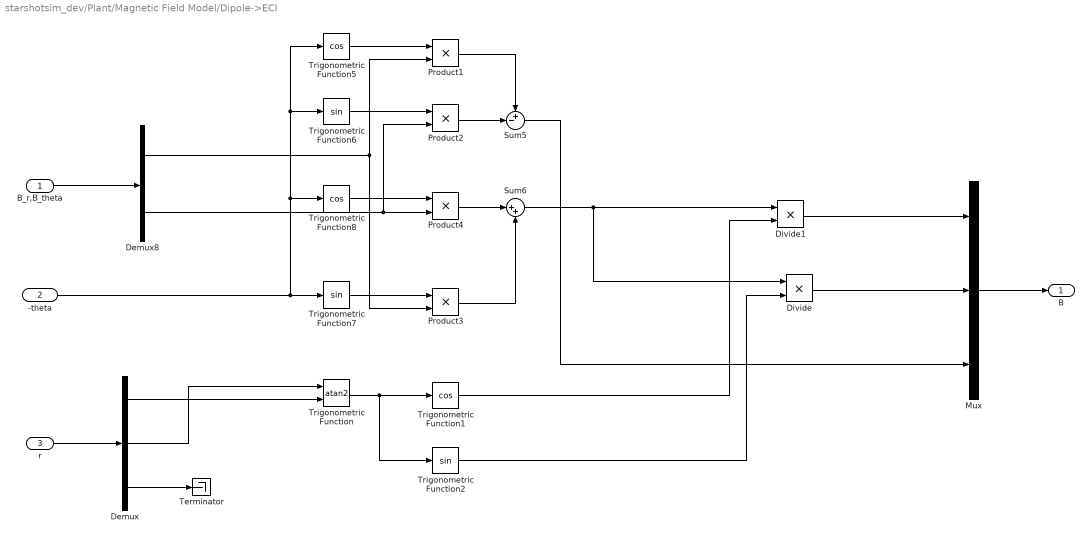
== system starshotsim_dev/Plant/Magnetic Field Model/Dipole->ECI ==
  B_r,B_theta : Inport
  -theta : Inport  Port=2
  r : Inport  Port=3
  Demux : Demux  Outputs=3
  Demux8 : Demux  Outputs=2
  Divide : Product  Inputs=**
  Divide1 : Product  Inputs=**
  Mux : Mux  Inputs=3
  Product{1..4} (4 alike) : Product
  Sum5 : Sum  Inputs=+-|
  Sum6 : Sum  Inputs=|++
  Terminator : Terminator
  Trigonometric Function : Trigonometry  Operator=atan2
  Trigonometric Function1 : Trigonometry  Operator=cos
  Trigonometric Function2 : Trigonometry
  Trigonometric Function5 : Trigonometry  Operator=cos
  Trigonometric Function6 : Trigonometry
  Trigonometric Function7 : Trigonometry
  Trigonometric Function8 : Trigonometry  Operator=cos
  B : Outport
  wires:
  -theta/1 -> Trigonometric Function5/1, Trigonometric Function6/1, Trigonometric Function8/1, Trigonometric Function7/1
  Product4/1 -> Sum6/1
  Product3/1 -> Sum6/2
  Demux8/1 -> Product3/2, Product1/2
  Demux8/2 -> Product2/2, Product4/2
  Trigonometric Function5/1 -> Product1/1
  Product2/1 -> Sum5/2
  Trigonometric Function7/1 -> Product3/1
  B_r,B_theta/1 -> Demux8/1
  Sum5/1 -> Mux/3
  Trigonometric Function8/1 -> Product4/1
  Trigonometric Function6/1 -> Product2/1
  Sum6/1 -> Divide1/1, Divide/1
  Product1/1 -> Sum5/1
  r/1 -> Demux/1
  Demux/3 -> Terminator/1
  Demux/2 -> Trigonometric Function/1
  Demux/1 -> Trigonometric Function/2
  Trigonometric Function/1 -> Trigonometric Function1/1, Trigonometric Function2/1
  Trigonometric Function1/1 -> Divide1/2
  Trigonometric Function2/1 -> Divide/2
  Mux/1 -> B/1
  Divide1/1 -> Mux/1
  Divide/1 -> Mux/2

== system starshotsim_dev/Plant/Quaternion Integration/q_normalize ==
  q_in : Inport  PortDimensions=4
  Dot Product : DotProduct  OutDataTypeStr=Inherit: Inherit via internal rule
  Math Function : Math  Operator=sqrt  SignedPower=on
  Product : Product  Inputs=*/  InputSameDT=on  SaturateOnIntegerOverflow=on  OutDataTypeStr=Inherit: Same as first input
  q_out : Outport
  wires:
  Product/1 -> q_out/1
  Math Function/1 -> Product/2
  Dot Product/1 -> Math Function/1
  q_in/1 -> Dot Product/2, Dot Product/1, Product/1

== system starshotsim_dev/Plant/Quaternion Integration/qderiv ==
  w : Inport
  q : Inport  Port=2
  Mux : Mux  Inputs=2
  Mux1 : Mux
  qd1 : Fcn  Expr=(u(7)*u(1)-u(6)*u(2)+u(5)*u(3))/2
  qd2 : Fcn  Expr=(u(6)*u(1)+u(7)*u(2)-u(4)*u(3))/2
  qd3 : Fcn  Expr=(-u(5)*u(1)+u(4)*u(2)+u(7)*u(3))/2
  qd4 : Fcn  Expr=(-u(4)*u(1)-u(5)*u(2)-u(6)*u(3))/2
  qd : Outport
  wires:
  Mux1/1 -> qd/1
  qd4/1 -> Mux1/4
  qd3/1 -> Mux1/3
  qd2/1 -> Mux1/2
  qd1/1 -> Mux1/1
  Mux/1 -> qd4/1, qd3/1, qd2/1, qd1/1
  q/1 -> Mux/2
  w/1 -> Mux/1

== system starshotsim_dev/Plant/qtoQ/Subsystem ==
  In1 : Inport
  3x3 : Reshape  OutputDimensionality=Customize  OutputDimensions=[3,3]
  Demux : Demux  Outputs=3
      settings: DisplayOption=none
  Gain : Gain  Gain=-1  SaturateOnIntegerOverflow=on  OutDataTypeStr=Inherit: Same as input  ParamDataTypeStr=Inherit: Same as input
  Gain1 : Gain  Gain=-1  SaturateOnIntegerOverflow=on  OutDataTypeStr=Inherit: Same as input  ParamDataTypeStr=Inherit: Same as input
  Gain2 : Gain  Gain=-1  SaturateOnIntegerOverflow=on  OutDataTypeStr=Inherit: Same as input  ParamDataTypeStr=Inherit: Same as input
  Mux : Mux  Inputs=9
  "diag 0 " : Constant  Value=0
  Out1 : Outport
  wires:
  Gain2/1 -> Mux/8
  Demux/1 -> Gain2/1, Mux/6
  Gain1/1 -> Mux/4
  Demux/2 -> Mux/7, Gain/1
  Gain/1 -> Mux/3
  Demux/3 -> Gain1/1, Mux/2
  Mux/1 -> 3x3/1
  "diag 0 "/1 -> Mux/9, Mux/5, Mux/1
  3x3/1 -> Out1/1
  In1/1 -> Demux/1

== system starshotsim_dev/Plant/qtoQ1/Subsystem ==
  In1 : Inport
  3x3 : Reshape  OutputDimensionality=Customize  OutputDimensions=[3,3]
  Demux : Demux  Outputs=3
      settings: DisplayOption=none
  Gain : Gain  Gain=-1  SaturateOnIntegerOverflow=on  OutDataTypeStr=Inherit: Same as input  ParamDataTypeStr=Inherit: Same as input
  Gain1 : Gain  Gain=-1  SaturateOnIntegerOverflow=on  OutDataTypeStr=Inherit: Same as input  ParamDataTypeStr=Inherit: Same as input
  Gain2 : Gain  Gain=-1  SaturateOnIntegerOverflow=on  OutDataTypeStr=Inherit: Same as input  ParamDataTypeStr=Inherit: Same as input
  Mux : Mux  Inputs=9
  "diag 0 " : Constant  Value=0
  Out1 : Outport
  wires:
  In1/1 -> Demux/1
  3x3/1 -> Out1/1
  "diag 0 "/1 -> Mux/1, Mux/5, Mux/9
  Mux/1 -> 3x3/1
  Demux/3 -> Mux/2, Gain1/1
  Gain/1 -> Mux/3
  Demux/2 -> Gain/1, Mux/7
  Gain1/1 -> Mux/4
  Demux/1 -> Mux/6, Gain2/1
  Gain2/1 -> Mux/8

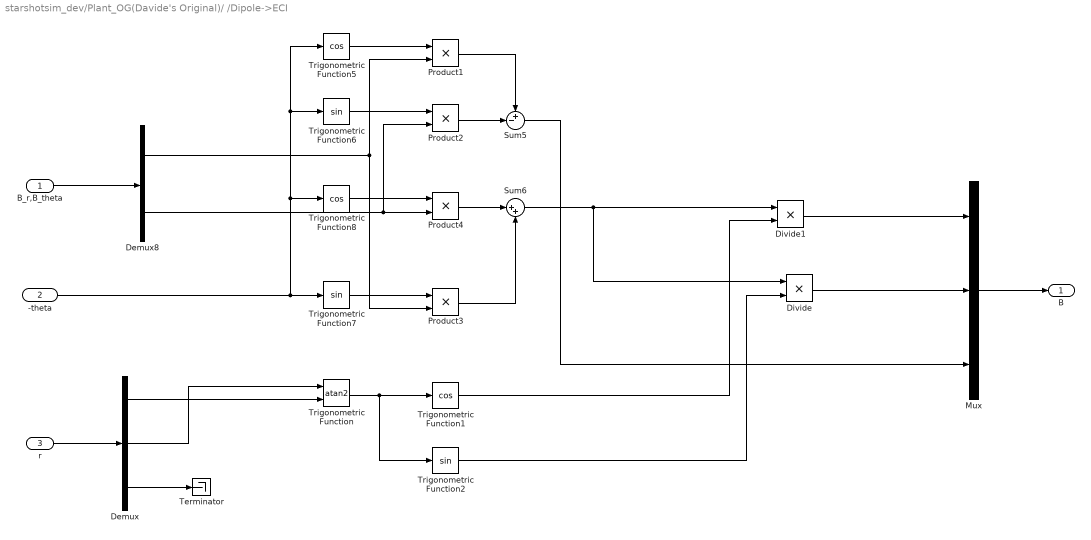
== system starshotsim_dev/Plant_OG(Davide's Original)/ /Dipole->ECI ==
  B_r,B_theta : Inport
  -theta : Inport  Port=2
  r : Inport  Port=3
  Demux : Demux  Outputs=3
  Demux8 : Demux  Outputs=2
  Divide : Product  Inputs=**
  Divide1 : Product  Inputs=**
  Mux : Mux  Inputs=3
  Product{1..4} (4 alike) : Product
  Sum5 : Sum  Inputs=+-|
  Sum6 : Sum  Inputs=|++
  Terminator : Terminator
  Trigonometric Function : Trigonometry  Operator=atan2
  Trigonometric Function1 : Trigonometry  Operator=cos
  Trigonometric Function2 : Trigonometry
  Trigonometric Function5 : Trigonometry  Operator=cos
  Trigonometric Function6 : Trigonometry
  Trigonometric Function7 : Trigonometry
  Trigonometric Function8 : Trigonometry  Operator=cos
  B : Outport
  wires:
  -theta/1 -> Trigonometric Function5/1, Trigonometric Function6/1, Trigonometric Function8/1, Trigonometric Function7/1
  Product4/1 -> Sum6/1
  Product3/1 -> Sum6/2
  Demux8/1 -> Product3/2, Product1/2
  Demux8/2 -> Product2/2, Product4/2
  Trigonometric Function5/1 -> Product1/1
  Product2/1 -> Sum5/2
  Trigonometric Function7/1 -> Product3/1
  B_r,B_theta/1 -> Demux8/1
  Sum5/1 -> Mux/3
  Trigonometric Function8/1 -> Product4/1
  Trigonometric Function6/1 -> Product2/1
  Sum6/1 -> Divide1/1, Divide/1
  Product1/1 -> Sum5/1
  r/1 -> Demux/1
  Demux/3 -> Terminator/1
  Demux/2 -> Trigonometric Function/1
  Demux/1 -> Trigonometric Function/2
  Trigonometric Function/1 -> Trigonometric Function1/1, Trigonometric Function2/1
  Trigonometric Function1/1 -> Divide1/2
  Trigonometric Function2/1 -> Divide/2
  Mux/1 -> B/1
  Divide1/1 -> Mux/1
  Divide/1 -> Mux/2

== system starshotsim_dev/Plant_OG(Davide's Original)/   /Normalized quat ==
  q : Inport
  Modulo1 : Subsystem
  Product2 : Product  Inputs=*/  SaturateOnIntegerOverflow=on  OutDataTypeStr=Inherit: Same as first input
  q^ : Outport
  wires:
  q/1 -> Modulo1/1(q), Product2/1
  Modulo1/1(Module q) -> Product2/2
  Product2/1 -> q^/1

== system starshotsim_dev/Plant_OG(Davide's Original)/     /(w_b)x(L_b) ==
  w_b : Inport
  L_b : Inport  Port=2
  Demux : Demux  Outputs=3
  Demux1 : Demux  Outputs=3
  Inv(I) : Gain  Gain=starshot.IC.massproperties.I  Multiplication=Matrix(K*u)
  Mux : Mux  Inputs=3
  Product{,1..5} (6 alike) : Product
  Sum : Sum  Inputs=+|-
  Sum1 : Sum  Inputs=-|+
  Sum2 : Sum  Inputs=+|-
  (w_b)x(L_b) : Outport
  wires:
  w_b/1 -> Demux/1
  L_b/1 -> Inv(I)/1
  Demux/3 -> Product1/1, Product3/1  "w_3"
  Demux/2 -> Product5/1, Product/1  "w_2"
  Demux/1 -> Product2/1, Product4/1  "w_1"
  Mux/1 -> (w_b)x(L_b)/1
  Demux1/3 -> Product2/2, Product/2  "L_3"
  Demux1/2 -> Product1/2, Product4/2  "L_2"
  Product1/1 -> Sum/2
  Product/1 -> Sum/1
  Demux1/1 -> Product5/2, Product3/2  "L_1"
  Sum/1 -> Mux/1
  Sum2/1 -> Mux/3
  Sum1/1 -> Mux/2
  Product5/1 -> Sum2/2
  Product4/1 -> Sum2/1
  Product3/1 -> Sum1/2
  Product2/1 -> Sum1/1
  Inv(I)/1 -> Demux1/1

== system starshotsim_dev/Plant_OG(Davide's Original)/quat to DCM/Subsystem ==
  In1 : Inport
  3x3 : Reshape  OutputDimensionality=Customize  OutputDimensions=[3,3]
  Demux : Demux  Outputs=3
      settings: DisplayOption=none
  Gain : Gain  Gain=-1  SaturateOnIntegerOverflow=on  OutDataTypeStr=Inherit: Same as input  ParamDataTypeStr=Inherit: Same as input
  Gain1 : Gain  Gain=-1  SaturateOnIntegerOverflow=on  OutDataTypeStr=Inherit: Same as input  ParamDataTypeStr=Inherit: Same as input
  Gain2 : Gain  Gain=-1  SaturateOnIntegerOverflow=on  OutDataTypeStr=Inherit: Same as input  ParamDataTypeStr=Inherit: Same as input
  Mux : Mux  Inputs=9
  "diag 0 " : Constant  Value=0
  Out1 : Outport
  wires:
  Gain2/1 -> Mux/8
  Demux/1 -> Gain2/1, Mux/6
  Gain1/1 -> Mux/4
  Demux/2 -> Mux/7, Gain/1
  Gain/1 -> Mux/3
  Demux/3 -> Gain1/1, Mux/2
  Mux/1 -> 3x3/1
  "diag 0 "/1 -> Mux/9, Mux/5, Mux/1
  3x3/1 -> Out1/1
  In1/1 -> Demux/1

== system starshotsim_dev/StarshotACS/KD_controller/Cross ==
  A : Inport
  B : Inport  Port=2
  Mux4 : Mux  Inputs=3
  Product{,1..5} (6 alike) : Product  InputSameDT=on  SaturateOnIntegerOverflow=on  OutDataTypeStr=Inherit: Same as first input
  Sum : Sum  Inputs=+-  InputSameDT=on  SaturateOnIntegerOverflow=on  OutDataTypeStr=Inherit: Same as first input
  Sum1 : Sum  Inputs=+-  InputSameDT=on  SaturateOnIntegerOverflow=on  OutDataTypeStr=Inherit: Same as first input
  Sum2 : Sum  Inputs=+-  InputSameDT=on  SaturateOnIntegerOverflow=on  OutDataTypeStr=Inherit: Same as first input
  demux2 : Demux  Outputs=3
      settings: DisplayOption=none
  demux3 : Demux  Outputs=3
      settings: DisplayOption=none
  AxB : Outport  InitialOutput=0
  wires:
  A/1 -> demux2/1
  B/1 -> demux3/1
  demux2/3 -> Product1/1, Product2/1
  demux3/3 -> Product/2, Product3/2
  demux2/1 -> Product3/1, Product4/1
  demux3/2 -> Product1/2, Product4/2
  demux2/2 -> Product/1, Product5/1
  demux3/1 -> Product2/2, Product5/2
  Product/1 -> Sum/1
  Product1/1 -> Sum/2
  Product2/1 -> Sum1/1
  Product3/1 -> Sum1/2
  Product4/1 -> Sum2/1
  Product5/1 -> Sum2/2
  Sum/1 -> Mux4/1
  Sum1/1 -> Mux4/2
  Sum2/1 -> Mux4/3
  Mux4/1 -> AxB/1

== system starshotsim_dev/StarshotACS/KD_controller/Skew matrix S(m)1 ==
  w : Inport
  Constant3 : Constant  Value=0
  Demux : Demux  Outputs=3
  Gain : Gain  Gain=-1
  Gain1 : Gain  Gain=-1
  Gain2 : Gain  Gain=-1
  Mux : Mux  Inputs=3
  Mux1 : Mux  Inputs=3
  Mux2 : Mux  Inputs=3
  Vector Concatenate : Concatenate  NumInputs=3  Mode=Multidimensional array  ConcatenateDimension=2
  S(w) : Outport
  wires:
  Gain/1 -> Mux/3
  Demux/2 -> Mux2/1, Gain/1
  Demux/3 -> Gain1/1, Mux/2
  Gain2/1 -> Mux2/2
  Demux/1 -> Mux1/3, Gain2/1
  Mux1/1 -> Vector Concatenate/2
  w/1 -> Demux/1
  Constant3/1 -> Mux2/3, Mux/1, Mux1/2
  Vector Concatenate/1 -> S(w)/1
  Mux/1 -> Vector Concatenate/1
  Mux2/1 -> Vector Concatenate/3
  Gain1/1 -> Mux1/1

== system starshotsim_dev/StarshotACS/Orientation controller/Norm2 ==
  v : Inport
  Dot Product6 : DotProduct  OutDataTypeStr=Inherit: Inherit via internal rule
  Sqrt4 : Sqrt
  norm(v) : Outport
  wires:
  v/1 -> Dot Product6/1, Dot Product6/2
  Dot Product6/1 -> Sqrt4/1
  Sqrt4/1 -> norm(v)/1

== system starshotsim_dev/StarshotACS/Orientation controller/Norm3 ==
  v : Inport
  Dot Product6 : DotProduct  OutDataTypeStr=Inherit: Inherit via internal rule
  Sqrt4 : Sqrt
  norm(v) : Outport
  wires:
  v/1 -> Dot Product6/1, Dot Product6/2
  Dot Product6/1 -> Sqrt4/1
  Sqrt4/1 -> norm(v)/1

== system starshotsim_dev/StarshotACS/Orientation controller/Skew matrix S(tau_c)1 ==
  omega : Inport
  Constant3 : Constant  Value=0
  Demux : Demux  Outputs=3
  Gain : Gain  Gain=-1
  Gain1 : Gain  Gain=-1
  Gain2 : Gain  Gain=-1
  Mux : Mux  Inputs=3
  Mux1 : Mux  Inputs=3
  Mux2 : Mux  Inputs=3
  Vector Concatenate : Concatenate  NumInputs=3  Mode=Multidimensional array  ConcatenateDimension=2
  S(omega) : Outport
  wires:
  Gain/1 -> Mux/3
  Demux/2 -> Mux2/1, Gain/1  "2"
  Demux/3 -> Gain1/1, Mux/2  "3"
  Gain2/1 -> Mux2/2
  Demux/1 -> Mux1/3, Gain2/1  "1"
  Mux1/1 -> Vector Concatenate/2
  omega/1 -> Demux/1
  Constant3/1 -> Mux2/3, Mux/1, Mux1/2  "0"
  Vector Concatenate/1 -> S(omega)/1
  Mux/1 -> Vector Concatenate/1
  Mux2/1 -> Vector Concatenate/3
  Gain1/1 -> Mux1/1
